simulink model "InbuiltDynamicsModelTest"  (R2024b)
settings: Solver=VariableStepAuto  StartTime=0.0  StopTime=inf  RelTol=1e-3
undefined symbols (not defined in the file or in its folder): omega, sat
libraries: aerolibutil x1, simulink_extras x1, sharedtransform x1
settings Model: Creator=Ameya  LastModifiedBy=Ameya

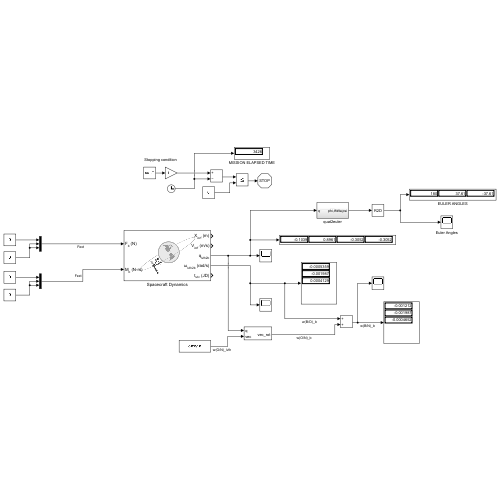
[thumbnail: Simulink's stored preview of the top-level diagram]
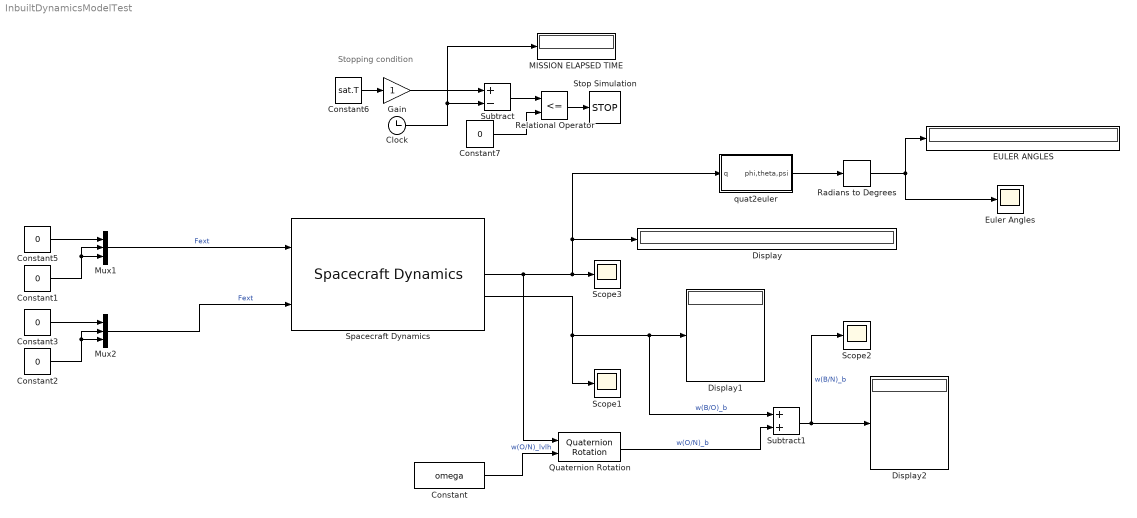
== system InbuiltDynamicsModelTest ==
  note: Stopping condition
  Clock : Clock
  Constant : Constant  Value=omega
  Constant{1..3,5,7} (5 alike) : Constant  Value=0
  Constant6 : Constant  Value=sat.T
  Display : Display
  Display1 : Display
  Display2 : Display
  EULER ANGLES : Display
  Euler Angles : Scope
  Gain : Gain
  MISSION ELAPSED TIME : Display
  Mux1 : Mux  Inputs=3
  Mux2 : Mux  Inputs=3
  Quaternion Rotation : aerolibutil/Quaternion Rotation
  Radians to Degrees : simulink_extras/Transformations/Radians to Degrees
  Relational Operator : RelationalOperator  Operator=<=  OutDataTypeStr=boolean  RndMeth=Simplest  InputSameDT=off
  Scope1 : Scope
  Scope2 : Scope
  Scope3 : Scope
  Spacecraft Dynamics : SpacecraftDynamics  mass=sat.mass  inertia=sat.J  semiMajorAxis=sat.a  eccentricity=sat.e  inclination=sat.i  raan=sat.RAAN  argPeriapsis=sat.w  trueAnomaly=sat.ta  attitudeFrame=LVLH  attitude=[1;0;0;0]  attitudeRate=sat.omegaBO  useGravGrad=off  gravityModel=Point-mass  angleUnits=Radians
  Stop Simulation : Stop
  Subtract : Sum  Inputs=+-
  Subtract1 : Sum
  quat2euler : Subsystem
  wires:
  Constant5/1 -> Mux1/1
  Constant1/1 -> Mux1/2, Mux1/3
  Mux1/1 -> Spacecraft Dynamics/1  "Fext"
  Spacecraft Dynamics/3 -> Quaternion Rotation/1, Scope3/1, Display/1, quat2euler/1(q)
  Spacecraft Dynamics/4 -> Scope1/1, Subtract1/1, Display1/1  "w(B/O)_b"
  Constant6/1 -> Gain/1
  Clock/1 -> MISSION ELAPSED TIME/1, Subtract/2
  Subtract/1 -> Relational Operator/1
  Relational Operator/1 -> Stop Simulation/1
  Gain/1 -> Subtract/1
  Constant7/1 -> Relational Operator/2
  Mux2/1 -> Spacecraft Dynamics/2  "Fext"
  Constant3/1 -> Mux2/1
  Constant2/1 -> Mux2/2, Mux2/3
  Quaternion Rotation/1 -> Subtract1/2  "w(O/N)_b"
  Constant/1 -> Quaternion Rotation/2  "w(O/N)_lvlh"
  Subtract1/1 -> Scope2/1, Display2/1  "w(B/N)_b"
  Radians to Degrees/1 -> Euler Angles/1, EULER ANGLES/1
  quat2euler/1(phi,theta,psi) -> Radians to Degrees/1

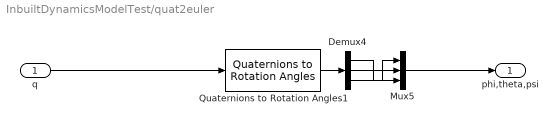
== system InbuiltDynamicsModelTest/quat2euler ==
  q : Inport
  Demux4 : Demux  Outputs=3
  Mux5 : Mux  Inputs=3
  Quaternions to Rotation Angles1 : sharedtransform/Quaternions to Rotation Angles  rotationOrder=ZYX  aMode=aMode
  phi,theta,psi : Outport
  wires:
  Quaternions to Rotation Angles1/1 -> Demux4/1
  Demux4/3 -> Mux5/1
  Demux4/2 -> Mux5/2
  Demux4/1 -> Mux5/3
  q/1 -> Quaternions to Rotation Angles1/1
  Mux5/1 -> phi,theta,psi/1
